simulink model "lftModel"  (R2024a)
settings: Solver=ode1  StartTime=0.0  StopTime=Inf  FixedStep=0.001  RelTol=1e-3
PostLoadFcn:
  | , if any(exist('dsrtsu_mdlpostloadfcn', 'file') ~= 0), dsrtsu_mdlpostloadfcn('Execute', bdroot); end,
InitFcn:
  | , if any(exist('rtifpga_mdlclblib', 'file') ~= 0), rtifpga_mdlclblib('Init', bdroot); end,
undefined symbols (not defined in the file): ampN, Current_Limit, cycles, fb, ff, fHz, fIN, freqs, lc, lcam, Mag_xData, Mag_yData, trajData, wn, xData, yData, z_stroke, z_TDC
libraries: rti1202lib_adc_class1 x7, rti1202lib_dio_class1 x3, simulink x3, rti1202lib_dac_class1 x1
(part 4 of 4)

== matlab function lftModel/Sweep Test/MATLAB Function ==
  data: eStop input; bPush input; tIn input; y output size=1; x0 input size=3; x1 output size=3; freqs parameter; cycles parameter
function [y,x1] = fcn(eStop, bPush, tIn, x0, freqs, cycles)

  % Named index notation. The commented out ones are used in helper
  % functions. They are left here for reference.

  MODE = 1; % 0==OFF, 1==RUN
  % TS   = 2; % Start time for the current cycle, s
  % NC   = 3; % Current cycle number, #

  % RUN  = 1; % Used by MODE, sweep is running
  OFF  = 0; % Used by MODE, sweep is not running

  % Update states using a pass through, modify them below as needed
  x1 = x0;

  % If user pushes the 'Start Sweep" button in Control Desk and the sweep
  % is not running (tStart0 < 0) then latch the time when the button was
  % pressed, tStart1 = tIn. Since tStart1 is now > 0, the function knows
  % the sweep is running. Note: once the sweep starts, the only way to stop
  % it is with the Control Desk eStop Sweep button.
  if (x1(MODE) == OFF) && (bPush > 0.5)
    x1 = startSweep(tIn);
  end

  if (x1(MODE) == OFF) || (eStop > 0.5)
      [y,x1] = resetSweep(tIn);
  else % sweep is running
      if endOfCycle(x1,tIn,freqs,cycles) % switch to the next cycle
          if isLastCycle(x1,cycles)      % last cycle
              [y,x1] = resetSweep(tIn);  % done sweeping
          else
              x1 = nextCycle(x1,tIn);             % update cycle info
              y = nextSweepPoint(x1,tIn,freqs);   % calc y
          end
      else
          y = nextSweepPoint(x1,tIn,freqs); % calc y
      end
  end

end % DONE!!

% Helper Functions

function x = startSweep(t)
% STARTSWEEP sets the state for starting the sweep

  MODE = 1; % 0==OFF, 1==RUN
  TS   = 2; % Start time for the current cycle, s
  NC   = 3; % Current cycle number, #

  RUN  = 1; % Used by MODE, sweep is running

  % code gen requires output variable setting before subscripting
  x = zeros(3,1);

  x(MODE) = RUN; % running
  x(NC) = 1;     % first cycle #
  x(TS) = t;     % latch start time for first cycle

end

function y = endOfCycle(x,t,freqs,cycles) 
% ENDOFCYCLE returns true if the cycle is done

  TS   = 2; % Start time for the current cycle, s
  NC   = 3; % Current cycle number, #

  y = t - x(TS) >= cycles(x(NC)) / freqs(x(NC));
end

function y = isLastCycle(x,cycles)
% ISLASTCYLCE returns true if this is the last cycle

  NC   = 3; % Current cycle number, #

  y = x(NC) == length(cycles);
end

function x1 = nextCycle(x0,t)
% NEXTCYCLE updates state to start the next cycle

  TS   = 2; % Start time for the current cycle, s
  NC   = 3; % Current cycle number, #

  % code gen requires output variable setting before subscripting
  x1 = x0;
  x1(NC) = x1(NC) + 1;
  x1(TS) = t;
end

function [y,x1] = resetSweep(t)
% RESETSWEEP stop and be ready to run again if asked

  MODE = 1; % 0==OFF, 1==RUN
  TS   = 2; % Start time for the current cycle, s
  NC   = 3; % Current cycle number, #

  %RUN  = 1; % Used by MODE, sweep is running
  OFF  = 0; % Used by MODE, sweep is not running

  % code gen requires output variable setting before subscripting
  x1 = zeros(3,1);  

  x1(MODE) = OFF;
  x1(TS) = t;
  x1(NC) = 0;

  y = 0;
  
end

function y = nextSweepPoint(x1,tIn,freqs)
% NEXTSWEEPPOINT calculates the next value of the sweep output

  TS   = 2; % Start time for the current cycle, s
  NC   = 3; % Current cycle number, #
  amp = 0.5;
  y = amp*sin(2*pi*freqs(x1(NC))*(tIn-x1(TS)));

end

== matlab function lftModel/Feedforward/Traj/MATLAB Function ==
  data: time input size=1; buttonPress input size=1; stateOld input size=2; stateNew output size=2
function stateNew = onoffToggle(time,buttonPress,stateOld)
% ONOFFTOGGLE starts a sine wave when buttonPress goes high and turns it off
% when it goes low
%
% If the sine wave playState is OFF when the button is pressed, then the
% current time is latched, and the sine wave is started. If the button is
% pressed when the sine wave playState is ON, then time is reset to zero
% and the sine wave stops immediately.
%
% Truth table
%   buttonPress      playState     Action
%  ------------------------------------------------------------------------
%       0                0         timeState = 0
%                                  playState = 0
%                                  yOut = 0
%       0                1         timeState = 0
%                                  playState = 0
%                                  yOut = 0
%       1                0         timeState = time
%                                  playState = 1
%                                  yOut = sine(time-timeState)
%       1                1         timeState = no change
%                                  playState = no change
%                                  yOut = sine(time-timeState)

  % Set buttonPress to 0 or 1 despite what any user tries to do...
  if buttonPress < 0
      buttonPress = 0;
  end

  if buttonPress > 1
      buttonPress = 1;
  end

  % Extract a states
  timeStateOld = stateOld(2);
  playStateOld = stateOld(1);  

  % Init, default the output = 0, and the new states = old states
  timeStateNew = timeStateOld;
  playStateNew = playStateOld;

  % Implement truth table
  if ~buttonPress
      timeStateNew = 0;
      playStateNew = 0;
  elseif ~playStateOld
      timeStateNew = time;
      playStateNew = 1;
  end

  % Update state
  stateNew = [playStateNew; timeStateNew];

== matlab function lftModel/Feedforward/Sine Wave/MATLAB Function ==
  data: buttonPress input size=1; time input; stateOld input size=2; yOut output size=1; stateNew output size=2; ff parameter
function [yOut,stateNew] = sineToggle(buttonPress,time,stateOld,ff)
% SINETOGGLE starts a sine wave when buttonPress goes high and turns it off
% when it goes low
%
% If the sine wave playState is OFF when the button is pressed, then the
% current time is latched, and the sine wave is started. If the button is
% pressed when the sine wave playState is ON, then time is reset to zero
% and the sine wave stops immediately.
%
% Truth table
%   buttonPress      playState     Action
%  ------------------------------------------------------------------------
%       0                0         timeState = 0
%                                  playState = 0
%                                  yOut = 0
%       0                1         timeState = 0
%                                  playState = 0
%                                  yOut = 0
%       1                0         timeState = time
%                                  playState = 1
%                                  yOut = sine(time-timeState)
%       1                1         timeState = no change
%                                  playState = no change
%                                  yOut = sine(time-timeState)

  % Set buttonPress to 0 or 1 despite what any user tries to do...
  if buttonPress < 0
      buttonPress = 0;
  end

  if buttonPress > 1
      buttonPress = 1;
  end

  % Extract a states
  timeStateOld = stateOld(1);
  playStateOld = stateOld(2);  

  % Init, default the output = 0, and the new states = old states
  yOut = 0;
  timeStateNew = timeStateOld;
  playStateNew = playStateOld;

  % Extract sine settings
  w  = 2*pi*ff.f;  % frequency, r/s
  a  = ff.a;       % amplitude, units depend on application

  % Implement truth table
  if ~buttonPress
      timeStateNew = 0;
      playStateNew = 0;
      yOut = 0;
  elseif ~playStateOld
      timeStateNew = time;
      playStateNew = 1;
      yOut = a*sin(w*(time-timeStateNew));
  else
      yOut = a*sin(w*(time-timeStateNew));
  end


  % Update state
  stateNew = [timeStateNew; playStateNew];

== matlab function lftModel/Feedforward/FTraj /MATLAB Function ==
  data: time input size=1; buttonPress input size=1; stateOld input size=2; stateNew output size=2
function stateNew = onoffToggle(time,buttonPress,stateOld)
% ONOFFTOGGLE starts a sine wave when buttonPress goes high and turns it off
% when it goes low
%
% If the sine wave playState is OFF when the button is pressed, then the
% current time is latched, and the sine wave is started. If the button is
% pressed when the sine wave playState is ON, then time is reset to zero
% and the sine wave stops immediately.
%
% Truth table
%   buttonPress      playState     Action
%  ------------------------------------------------------------------------
%       0                0         timeState = 0
%                                  playState = 0
%                                  yOut = 0
%       0                1         timeState = 0
%                                  playState = 0
%                                  yOut = 0
%       1                0         timeState = time
%                                  playState = 1
%                                  yOut = sine(time-timeState)
%       1                1         timeState = no change
%                                  playState = no change
%                                  yOut = sine(time-timeState)

  % Set buttonPress to 0 or 1 despite what any user tries to do...
  if buttonPress < 0
      buttonPress = 0;
  end

  if buttonPress > 1
      buttonPress = 1;
  end

  % Extract a states
  timeStateOld = stateOld(2);
  playStateOld = stateOld(1);  

  % Init, default the output = 0, and the new states = old states
  timeStateNew = timeStateOld;
  playStateNew = playStateOld;

  % Implement truth table
  if ~buttonPress
      timeStateNew = 0;
      playStateNew = 0;
  elseif ~playStateOld
      timeStateNew = time;
      playStateNew = 1;
  end

  % Update state
  stateNew = [playStateNew; timeStateNew];

== matlab function lftModel/Feedforward/Force White Noise /MATLAB Function ==
  data: time input size=1; buttonPress input size=1; stateOld input size=2; stateNew output size=2
function stateNew = onoffToggle(time,buttonPress,stateOld)
% ONOFFTOGGLE starts a sine wave when buttonPress goes high and turns it off
% when it goes low
%
% If the sine wave playState is OFF when the button is pressed, then the
% current time is latched, and the sine wave is started. If the button is
% pressed when the sine wave playState is ON, then time is reset to zero
% and the sine wave stops immediately.
%
% Truth table
%   buttonPress      playState     Action
%  ------------------------------------------------------------------------
%       0                0         timeState = 0
%                                  playState = 0
%                                  yOut = 0
%       0                1         timeState = 0
%                                  playState = 0
%                                  yOut = 0
%       1                0         timeState = time
%                                  playState = 1
%                                  yOut = sine(time-timeState)
%       1                1         timeState = no change
%                                  playState = no change
%                                  yOut = sine(time-timeState)

  % Set buttonPress to 0 or 1 despite what any user tries to do...
  if buttonPress < 0
      buttonPress = 0;
  end

  if buttonPress > 1
      buttonPress = 1;
  end

  % Extract a states
  timeStateOld = stateOld(2);
  playStateOld = stateOld(1);  

  % Init, default the output = 0, and the new states = old states
  timeStateNew = timeStateOld;
  playStateNew = playStateOld;

  % Implement truth table
  if ~buttonPress
      timeStateNew = 0;
      playStateNew = 0;
  elseif ~playStateOld
      timeStateNew = time;
      playStateNew = 1;
  end

  % Update state
  stateNew = [playStateNew; timeStateNew];

== matlab function lftModel/Feedforward/FTraj /MATLAB Function1 ==
  data: t input; y output; T parameter
function y = pincher(t,T)
% PINCHER outputs a ramp starting at t=0 and ending at t = T
  if t<0
    y = 0;
  elseif t<T
    y = t/T;
  else
      y = 1;
  end
end
